simulink model "mass_spring_damper"  (R2020a)
settings: Solver=VariableStepAuto  StartTime=0.0  StopTime=10.0  RelTol=1e-3
undefined symbols (not defined in the file): c, dxdt_init, F_0, F_1, k, m, t_step_F, x_init
settings Model: Creator=Dhanush Wagle  LastModifiedBy=Dhanush Wagle

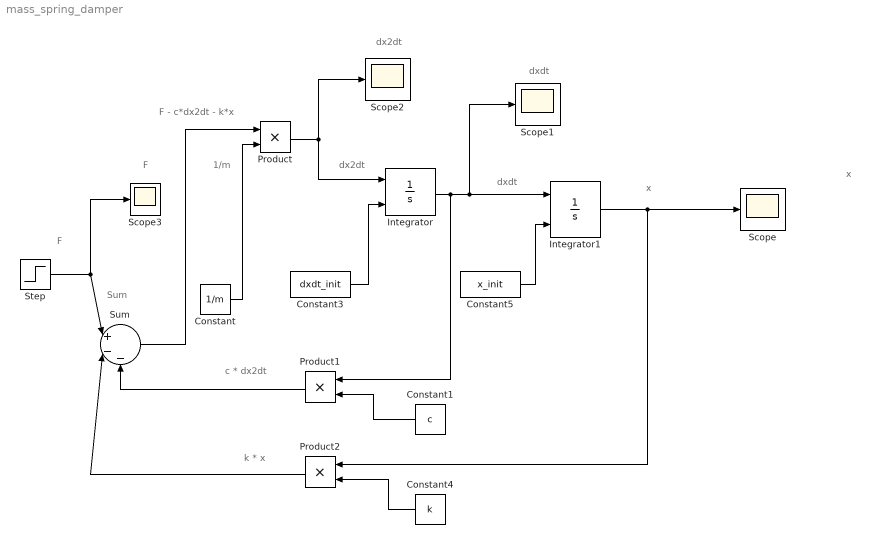
== system mass_spring_damper ==
  note: F
  note: x
  note: dxdt
  note: dx2dt
  note: 1/m
  note: F - c*dx2dt - k*x
  note: c * dx2dt
  note: k * x
  note: x
  note: dxdt
  note: dx2dt
  note: Sum
  note: F
  Constant : Constant  Value=1/m
  Constant1 : Constant  Value=c
  Constant3 : Constant  Value=dxdt_init
  Constant4 : Constant  Value=k
  Constant5 : Constant  Value=x_init
  Integrator : Integrator  InitialConditionSource=external
  Integrator1 : Integrator  InitialConditionSource=external
  Product : Product
  Product1 : Product
  Product2 : Product
  Scope{,1..3} (4 alike) : Scope
  Step : Step  Time=t_step_F  Before=F_0  After=F_1  SampleTime=0
  Sum : Sum  Inputs=|+--
  wires:
  Integrator/1 -> Product1/1, Scope1/1, Integrator1/1
  Integrator1/1 -> Product2/1, Scope/1
  Constant5/1 -> Integrator1/2
  Constant3/1 -> Integrator/2
  Constant1/1 -> Product1/2
  Constant4/1 -> Product2/2
  Product1/1 -> Sum/3
  Product2/1 -> Sum/2
  Step/1 -> Scope3/1, Sum/1
  Sum/1 -> Product/1
  Constant/1 -> Product/2
  Product/1 -> Scope2/1, Integrator/1
